simulink model "motor_pi_10ms"  (R2018b)
settings: Solver=FixedStepAuto  StartTime=0.0  StopTime=1  FixedStep=Ts  RelTol=1e-3
values from neighbouring files (symbols this model uses):
  Ki_l_A = (4*Tl)/(Kl*sigma_A*sigma_A)    (= 1.91131498471)    [motor_para_10ms.m]
  Ki_l_B = (4*Tl)/(Kl*sigma_B*sigma_B)    (= 2.64541866396)    [motor_para_10ms.m]
  Ki_l_C = (4*Tl)/(Kl*sigma_C*sigma_C)    (= 3.39789330615)    [motor_para_10ms.m]
  Ki_r_A = (4*Tr)/(Kr*sigma_A*sigma_A)    (= 2.21712538226)    [motor_para_10ms.m]
  Ki_r_B = (4*Tr)/(Kr*sigma_B*sigma_B)    (= 3.06868565019)    [motor_para_10ms.m]
  Ki_r_C = (4*Tr)/(Kr*sigma_C*sigma_C)    (= 3.94155623513)    [motor_para_10ms.m]
  Kl = 6.54    [motor_para_10ms.m]
  Kp_l_A = (1/Kl)*(((4*Tl)/sigma_A)-1)    (= 0.229357798165)    [motor_para_10ms.m]
  Kp_l_B = (1/Kl)*(((4*Tl)/sigma_B)-1)    (= 0.296815974096)    [motor_para_10ms.m]
  Kp_l_C = (1/Kl)*(((4*Tl)/sigma_C)-1)    (= 0.356778797146)    [motor_para_10ms.m]
  Kp_r_A = (1/Kr)*(4*Tr/sigma_A-1)    (= 0.290519877676)    [motor_para_10ms.m]
  Kp_r_B = (1/Kr)*(4*Tr/sigma_B-1)    (= 0.368771361756)    [motor_para_10ms.m]
  Kp_r_C = (1/Kr)*(4*Tr/sigma_A-1)    (= 0.290519877676)    [motor_para_10ms.m]
  Kr = 6.54    [motor_para_10ms.m]
  Ll = 0.01    [motor_para_10ms.m]
  Lr = 0.01    [motor_para_10ms.m]
  p1 = -2*exp(-rho/(2*mu))*cos(sqrt(2*mu-1)*rho/2*mu)    [motor_para_10ms.m]
  p2 = exp(-rho/mu)    [motor_para_10ms.m]
  Tl = 0.125    [motor_para_10ms.m]
  Tr = 0.145    [motor_para_10ms.m]
  Ts = 0.01    [motor_para_10ms.m]
settings Model: Creator=kshat  LastModifiedBy=m152069
settings OptimizationCC: DefaultParameterBehavior=Inlined  UseDivisionForNetSlopeComputation=on  UseFloatMulNetSlope=on  InlineInvariantSignals=on  PassReuseOutputArgsAs=Individual arguments  ZeroExternalMemoryAtStartup=off  ZeroInternalMemoryAtStartup=off  NoFixptDivByZeroProtection=on  EfficientFloat2IntCast=on  LifeSpan=1  OptimizeBlockOrder=speed  DifferentSizesBufferReuse=on
settings DebuggingCC: ParameterTunabilityLossMsg=error  LibraryContextMissingDiagnostic=none
settings HardwareCC: ProdBitPerPointer=32  ProdBitPerSizeT=32  ProdBitPerPtrDiffT=32  ProdLargestAtomicInteger=Long  ProdWordSize=32  ProdLongLongMode=on  ProdHWDeviceType=ARM Compatible->ARM 9
settings SFSimCC: SimUseLocalCustomCode=off  MATLABDynamicMemAlloc=off
settings RTWCC: SystemTargetFile=ert.tlc  TemplateMakefile=ert_default_tmf  GenerateReport=on  RTWUseLocalCustomCode=off  IncludeHyperlinkInReport=on  LaunchReport=on  TargetLang=C++  GenerateTraceInfo=on  GenerateTraceReport=on  GenerateTraceReportSl=on  GenerateTraceReportSf=on  GenerateTraceReportEml=on
settings CodeAppCC: ForceParamTrailComments=on  IgnoreCustomStorageClasses=off  OperatorAnnotations=on  SimulinkDataObjDesc=on  SFDataObjDesc=on  CustomSymbolStrGlobalVar=rt$N$M  CustomSymbolStrType=$N$M  CustomSymbolStrFcn=$N$M$F  CustomSymbolStrMacro=$N$M  InsertBlockDesc=on
settings ERTTargetCC: TargetLangStandard=C++03 (ISO)  GenerateSampleERTMain=on  IncludeMdlTerminateFcn=off  CombineSignalStateStructs=on  MultiInstanceERTCode=on  CodeInterfacePackaging=C++ class  SupportComplex=off  SupportContinuousTime=on  InlinedParameterPlacement=NonHierarchical  RootIOFormat=Structure reference  ERTCustomFileTemplate=example_file_process.tlc  ERTFilePackagingFormat=CompactWithDataFile

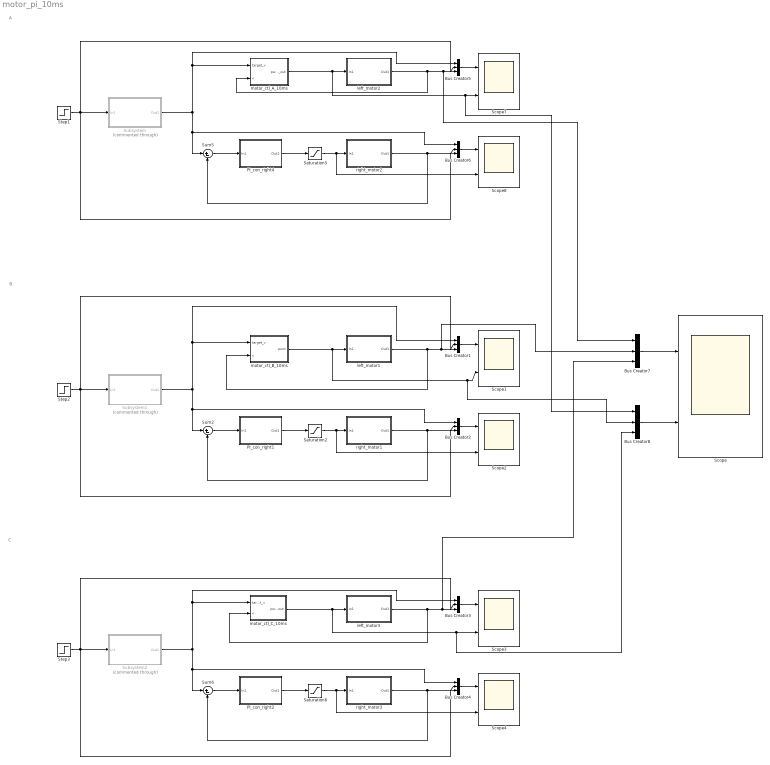
== system motor_pi_10ms ==
  note: C
  note: B
  note: A
  Bus Creator{1..8} (8 alike) : BusCreator  Inputs=3
  PI_con_right1 : Subsystem
  PI_con_right2 : Subsystem
  PI_con_right4 : Subsystem
  Saturation2 : Saturate  UpperLimit=100  LowerLimit=0
  Saturation5 : Saturate  UpperLimit=100  LowerLimit=0
  Saturation6 : Saturate  UpperLimit=100  LowerLimit=0
  Scope{,1..4,7..8} (7 alike) : Scope  NumInputPorts=2
  Step1 : Step  Time=0  After=400  SampleTime=0
  Step2 : Step  Time=0  After=400  SampleTime=0
  Step3 : Step  Time=0  After=400  SampleTime=0
  Subsystem : Subsystem  Commented=through
  Subsystem1 : Subsystem  Commented=through
  Subsystem2 : Subsystem  Commented=through
  Sum2 : Sum  Inputs=|+-
  Sum5 : Sum  Inputs=|+-
  Sum6 : Sum  Inputs=|+-
  left_motor1 : Subsystem
  left_motor2 : Subsystem
  left_motor3 : Subsystem
  motor_ctl_A_10ms : Subsystem  TreatAsAtomicUnit=on
  motor_ctl_B_10ms : Subsystem  TreatAsAtomicUnit=on
  motor_ctl_C_10ms : Subsystem
  right_motor1 : Subsystem
  right_motor2 : Subsystem
  right_motor3 : Subsystem
  wires:
  left_motor2/1(Out1) -> motor_ctl_A_10ms/2(v), Bus Creator7/1, Bus Creator5/2
  Sum5/1 -> PI_con_right4/1(In1)
  right_motor2/1(Out1) -> Sum5/2, Bus Creator6/2
  PI_con_right4/1(Out1) -> Saturation5/1
  Saturation5/1 -> Scope8/2, right_motor2/1(In1)
  Bus Creator6/1 -> Scope8/1
  Bus Creator5/1 -> Scope7/1
  Step1/1 -> Bus Creator6/3, Bus Creator5/3, Subsystem/1(In1)
  Subsystem/1(Out1) -> motor_ctl_A_10ms/1(target_v), Bus Creator5/1, Bus Creator6/1, Sum5/1
  left_motor1/1(Out1) -> motor_ctl_B_10ms/2(v), Bus Creator7/2, Bus Creator1/2
  PI_con_right1/1(Out1) -> Saturation2/1
  Sum2/1 -> PI_con_right1/1(In1)
  Saturation2/1 -> Scope2/2, right_motor1/1(In1)
  Step2/1 -> Bus Creator2/3, Bus Creator1/3, Subsystem1/1(In1)
  Subsystem1/1(Out1) -> motor_ctl_B_10ms/1(target_v), Bus Creator1/1, Bus Creator2/1, Sum2/1
  right_motor1/1(Out1) -> Sum2/2, Bus Creator2/2
  Bus Creator2/1 -> Scope2/1
  Bus Creator1/1 -> Scope1/1
  left_motor3/1(Out1) -> motor_ctl_C_10ms/2(v), Bus Creator7/3, Bus Creator3/2
  PI_con_right2/1(Out1) -> Saturation6/1
  Sum6/1 -> PI_con_right2/1(In1)
  Saturation6/1 -> Scope4/2, right_motor3/1(In1)
  Step3/1 -> Bus Creator4/3, Bus Creator3/3, Subsystem2/1(In1)
  Subsystem2/1(Out1) -> motor_ctl_C_10ms/1(target_v), Bus Creator3/1, Bus Creator4/1, Sum6/1
  right_motor3/1(Out1) -> Sum6/2, Bus Creator4/2
  Bus Creator4/1 -> Scope4/1
  Bus Creator3/1 -> Scope3/1
  Bus Creator7/1 -> Scope/1
  Bus Creator8/1 -> Scope/2
  motor_ctl_A_10ms/1(pwm_out) -> Bus Creator8/1, Scope7/2, left_motor2/1(In1)
  motor_ctl_B_10ms/1(pwm) -> Scope1/2, Bus Creator8/2, left_motor1/1(In1)
  motor_ctl_C_10ms/1(pwm_out) -> Bus Creator8/3, Scope3/2, left_motor3/1(In1)

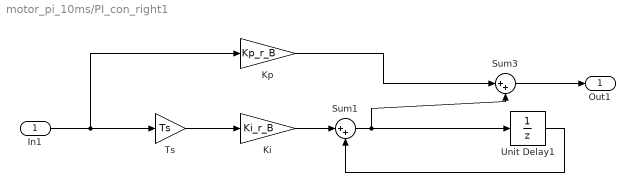
== system motor_pi_10ms/PI_con_right1 ==
  In1 : Inport
  Ki : Gain  Gain=Ki_r_B
  Kp : Gain  Gain=Kp_r_B
  Sum1 : Sum  Inputs=|++
  Sum3 : Sum  Inputs=|++
  Ts : Gain  Gain=Ts
  Unit Delay1 : UnitDelay  SampleTime=-1
  Out1 : Outport
  wires:
  Sum3/1 -> Out1/1
  Sum1/1 -> Unit Delay1/1, Sum3/2
  Ki/1 -> Sum1/1
  Kp/1 -> Sum3/1
  Ts/1 -> Ki/1
  Unit Delay1/1 -> Sum1/2
  In1/1 -> Kp/1, Ts/1

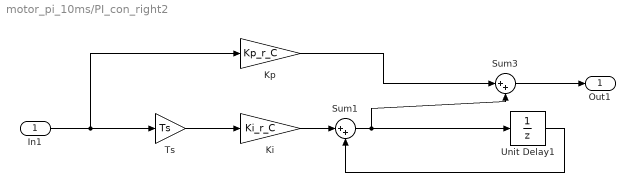
== system motor_pi_10ms/PI_con_right2 ==
  In1 : Inport
  Ki : Gain  Gain=Ki_r_C
  Kp : Gain  Gain=Kp_r_C
  Sum1 : Sum  Inputs=|++
  Sum3 : Sum  Inputs=|++
  Ts : Gain  Gain=Ts
  Unit Delay1 : UnitDelay  SampleTime=-1
  Out1 : Outport
  wires:
  Sum3/1 -> Out1/1
  Sum1/1 -> Unit Delay1/1, Sum3/2
  Ki/1 -> Sum1/1
  Kp/1 -> Sum3/1
  Ts/1 -> Ki/1
  Unit Delay1/1 -> Sum1/2
  In1/1 -> Kp/1, Ts/1

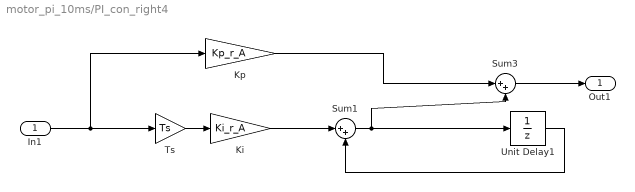
== system motor_pi_10ms/PI_con_right4 ==
  In1 : Inport
  Ki : Gain  Gain=Ki_r_A
  Kp : Gain  Gain=Kp_r_A
  Sum1 : Sum  Inputs=|++
  Sum3 : Sum  Inputs=|++
  Ts : Gain  Gain=Ts
  Unit Delay1 : UnitDelay  SampleTime=-1
  Out1 : Outport
  wires:
  Sum3/1 -> Out1/1
  Sum1/1 -> Unit Delay1/1, Sum3/2
  Ki/1 -> Sum1/1
  Kp/1 -> Sum3/1
  Ts/1 -> Ki/1
  Unit Delay1/1 -> Sum1/2
  In1/1 -> Kp/1, Ts/1

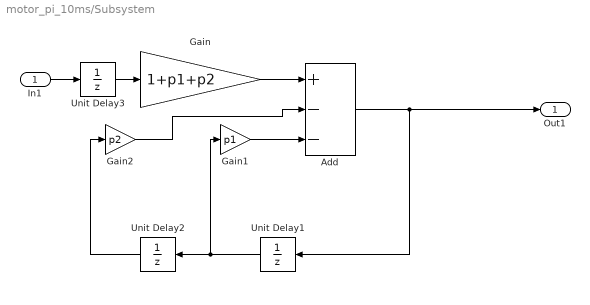
== system motor_pi_10ms/Subsystem ==
  In1 : Inport
  Add : Sum  Inputs=+--
  Gain : Gain  Gain=1+p1+p2
  Gain1 : Gain  Gain=p1
  Gain2 : Gain  Gain=p2
  Unit Delay1 : UnitDelay  SampleTime=-1
  Unit Delay2 : UnitDelay  SampleTime=-1
  Unit Delay3 : UnitDelay  SampleTime=-1
  Out1 : Outport
  wires:
  Unit Delay2/1 -> Gain2/1
  Unit Delay1/1 -> Gain1/1, Unit Delay2/1
  Unit Delay3/1 -> Gain/1
  Gain/1 -> Add/1
  Gain1/1 -> Add/3
  Gain2/1 -> Add/2
  Add/1 -> Out1/1, Unit Delay1/1
  In1/1 -> Unit Delay3/1

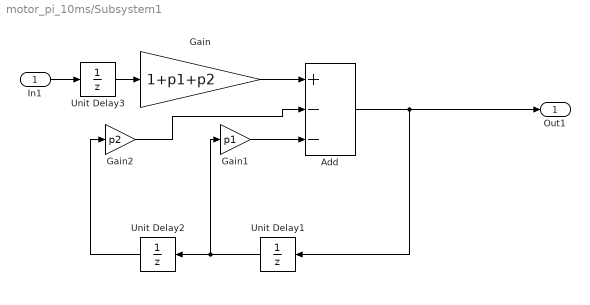
== system motor_pi_10ms/Subsystem1 ==
  In1 : Inport
  Add : Sum  Inputs=+--
  Gain : Gain  Gain=1+p1+p2
  Gain1 : Gain  Gain=p1
  Gain2 : Gain  Gain=p2
  Unit Delay1 : UnitDelay  SampleTime=-1
  Unit Delay2 : UnitDelay  SampleTime=-1
  Unit Delay3 : UnitDelay  SampleTime=-1
  Out1 : Outport
  wires:
  Unit Delay2/1 -> Gain2/1
  Unit Delay1/1 -> Gain1/1, Unit Delay2/1
  Unit Delay3/1 -> Gain/1
  Gain/1 -> Add/1
  Gain1/1 -> Add/3
  Gain2/1 -> Add/2
  Add/1 -> Out1/1, Unit Delay1/1
  In1/1 -> Unit Delay3/1

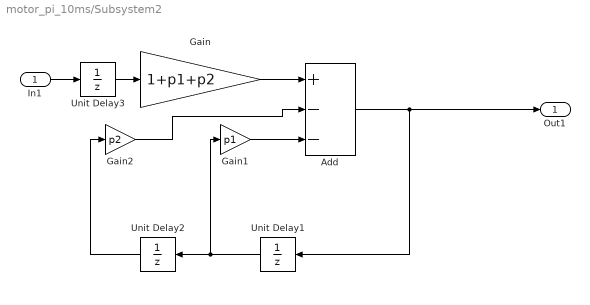
== system motor_pi_10ms/Subsystem2 ==
  In1 : Inport
  Add : Sum  Inputs=+--
  Gain : Gain  Gain=1+p1+p2
  Gain1 : Gain  Gain=p1
  Gain2 : Gain  Gain=p2
  Unit Delay1 : UnitDelay  SampleTime=-1
  Unit Delay2 : UnitDelay  SampleTime=-1
  Unit Delay3 : UnitDelay  SampleTime=-1
  Out1 : Outport
  wires:
  Unit Delay2/1 -> Gain2/1
  Unit Delay1/1 -> Gain1/1, Unit Delay2/1
  Unit Delay3/1 -> Gain/1
  Gain/1 -> Add/1
  Gain1/1 -> Add/3
  Gain2/1 -> Add/2
  Add/1 -> Out1/1, Unit Delay1/1
  In1/1 -> Unit Delay3/1

== system motor_pi_10ms/left_motor1 ==
  In1 : Inport
  Transfer Fcn : TransferFcn  Numerator=[Kl]  Denominator=[Tl 1]
  Transport Delay2 : TransportDelay  DelayTime=Ll
  Out1 : Outport
  wires:
  Transfer Fcn/1 -> Transport Delay2/1
  In1/1 -> Transfer Fcn/1
  Transport Delay2/1 -> Out1/1

== system motor_pi_10ms/left_motor2 ==
  In1 : Inport
  Transfer Fcn : TransferFcn  Numerator=[Kl]  Denominator=[Tl 1]
  Transport Delay2 : TransportDelay  DelayTime=Ll
  Out1 : Outport
  wires:
  Transfer Fcn/1 -> Transport Delay2/1
  In1/1 -> Transfer Fcn/1
  Transport Delay2/1 -> Out1/1

== system motor_pi_10ms/left_motor3 ==
  In1 : Inport
  Transfer Fcn : TransferFcn  Numerator=[Kl]  Denominator=[Tl 1]
  Transport Delay2 : TransportDelay  DelayTime=Ll
  Out1 : Outport
  wires:
  Transfer Fcn/1 -> Transport Delay2/1
  In1/1 -> Transfer Fcn/1
  Transport Delay2/1 -> Out1/1

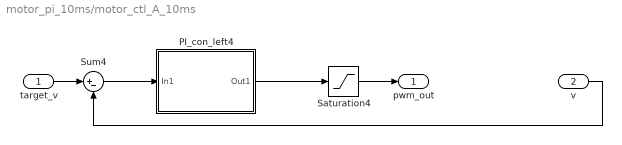
== system motor_pi_10ms/motor_ctl_A_10ms ==
  target_v : Inport
  v : Inport  Port=2
  PI_con_left4 : Subsystem
  Saturation4 : Saturate  UpperLimit=100  LowerLimit=0
  Sum4 : Sum  Inputs=|+-
  pwm_out : Outport
  wires:
  PI_con_left4/1(Out1) -> Saturation4/1
  Sum4/1 -> PI_con_left4/1(In1)
  v/1 -> Sum4/2
  Saturation4/1 -> pwm_out/1
  target_v/1 -> Sum4/1

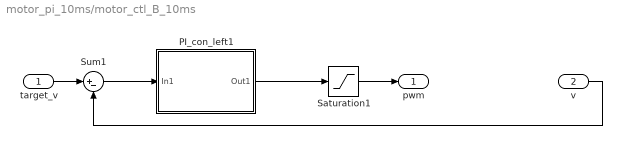
== system motor_pi_10ms/motor_ctl_B_10ms ==
  target_v : Inport
  v : Inport  Port=2
  PI_con_left1 : Subsystem
  Saturation1 : Saturate  UpperLimit=100  LowerLimit=0
  Sum1 : Sum  Inputs=|+-
  pwm : Outport
  wires:
  PI_con_left1/1(Out1) -> Saturation1/1
  v/1 -> Sum1/2
  Sum1/1 -> PI_con_left1/1(In1)
  Saturation1/1 -> pwm/1
  target_v/1 -> Sum1/1

== system motor_pi_10ms/motor_ctl_C_10ms ==
  target_v : Inport
  v : Inport  Port=2
  PI_con_left2 : Subsystem
  Saturation3 : Saturate  UpperLimit=100  LowerLimit=0
  Sum3 : Sum  Inputs=|+-
  pwm_out : Outport
  wires:
  PI_con_left2/1(Out1) -> Saturation3/1
  Sum3/1 -> PI_con_left2/1(In1)
  Saturation3/1 -> pwm_out/1
  v/1 -> Sum3/2
  target_v/1 -> Sum3/1

== system motor_pi_10ms/right_motor1 ==
  In1 : Inport
  Transfer Fcn1 : TransferFcn  Numerator=[Kr]  Denominator=[Tr 1]
  Transport Delay2 : TransportDelay  DelayTime=Lr
  Out1 : Outport
  wires:
  Transport Delay2/1 -> Out1/1
  In1/1 -> Transfer Fcn1/1
  Transfer Fcn1/1 -> Transport Delay2/1

== system motor_pi_10ms/right_motor2 ==
  In1 : Inport
  Transfer Fcn1 : TransferFcn  Numerator=[Kr]  Denominator=[Tr 1]
  Transport Delay2 : TransportDelay  DelayTime=Lr
  Out1 : Outport
  wires:
  Transport Delay2/1 -> Out1/1
  In1/1 -> Transfer Fcn1/1
  Transfer Fcn1/1 -> Transport Delay2/1

== system motor_pi_10ms/right_motor3 ==
  In1 : Inport
  Transfer Fcn1 : TransferFcn  Numerator=[Kr]  Denominator=[Tr 1]
  Transport Delay2 : TransportDelay  DelayTime=Lr
  Out1 : Outport
  wires:
  Transport Delay2/1 -> Out1/1
  In1/1 -> Transfer Fcn1/1
  Transfer Fcn1/1 -> Transport Delay2/1

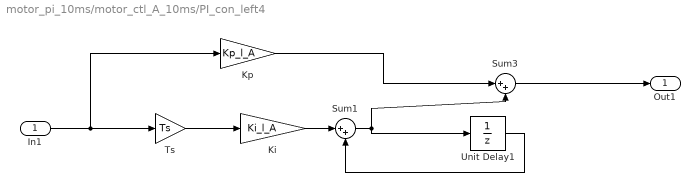
== system motor_pi_10ms/motor_ctl_A_10ms/PI_con_left4 ==
  In1 : Inport
  Ki : Gain  Gain=Ki_l_A
  Kp : Gain  Gain=Kp_l_A
  Sum1 : Sum  Inputs=|++
  Sum3 : Sum  Inputs=|++
  Ts : Gain  Gain=Ts
  Unit Delay1 : UnitDelay  SampleTime=-1
  Out1 : Outport
  wires:
  In1/1 -> Ts/1, Kp/1
  Unit Delay1/1 -> Sum1/2
  Ts/1 -> Ki/1
  Kp/1 -> Sum3/1
  Ki/1 -> Sum1/1
  Sum1/1 -> Sum3/2, Unit Delay1/1
  Sum3/1 -> Out1/1

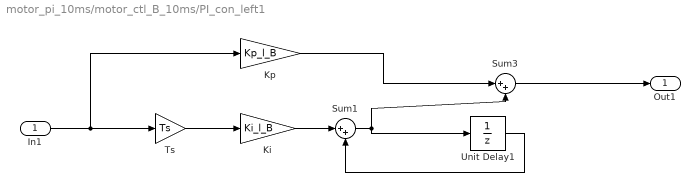
== system motor_pi_10ms/motor_ctl_B_10ms/PI_con_left1 ==
  In1 : Inport
  Ki : Gain  Gain=Ki_l_B
  Kp : Gain  Gain=Kp_l_B
  Sum1 : Sum  Inputs=|++
  Sum3 : Sum  Inputs=|++
  Ts : Gain  Gain=Ts
  Unit Delay1 : UnitDelay  SampleTime=-1
  Out1 : Outport
  wires:
  In1/1 -> Ts/1, Kp/1
  Unit Delay1/1 -> Sum1/2
  Ts/1 -> Ki/1
  Kp/1 -> Sum3/1
  Ki/1 -> Sum1/1
  Sum1/1 -> Sum3/2, Unit Delay1/1
  Sum3/1 -> Out1/1

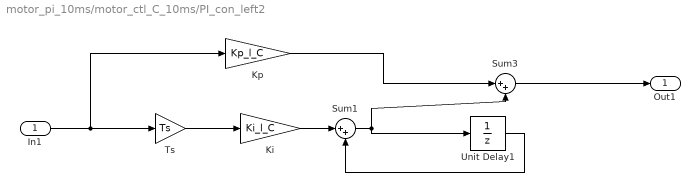
== system motor_pi_10ms/motor_ctl_C_10ms/PI_con_left2 ==
  In1 : Inport
  Ki : Gain  Gain=Ki_l_C
  Kp : Gain  Gain=Kp_l_C
  Sum1 : Sum  Inputs=|++
  Sum3 : Sum  Inputs=|++
  Ts : Gain  Gain=Ts
  Unit Delay1 : UnitDelay  SampleTime=-1
  Out1 : Outport
  wires:
  In1/1 -> Ts/1, Kp/1
  Unit Delay1/1 -> Sum1/2
  Ts/1 -> Ki/1
  Kp/1 -> Sum3/1
  Ki/1 -> Sum1/1
  Sum1/1 -> Sum3/2, Unit Delay1/1
  Sum3/1 -> Out1/1
